simulink model "test_track1"  (R2023a)
settings: Solver=VariableStepAuto  StartTime=0.0  StopTime=600  RelTol=1e-3
settings Model: Creator=lpb10197  LastModifiedBy=lpb10197
settings DebuggingCC: UnconnectedInputMsg=warning  UnconnectedOutputMsg=warning  UnconnectedLineMsg=warning
settings ModelReferenceCC: EnableRefExpFcnMdlSchedulingChecks=on
settings RTWCC: DLArmComputeVersion=19.05

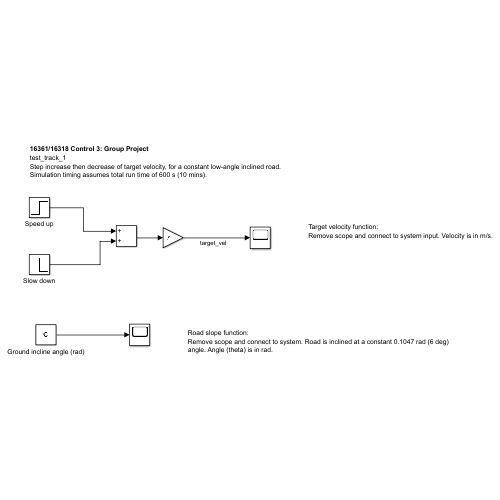
[thumbnail: Simulink's stored preview of the top-level diagram]
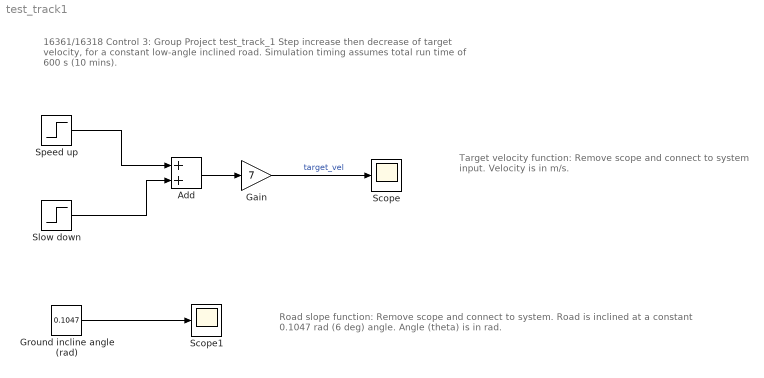
== system test_track1 ==
  note: Road slope function:
      | Remove scope and connect to system. Road is inclined at a constant 0.1047 rad (6 deg) angle. Angle (theta) is in rad.
  note: Target velocity function:
      | Remove scope and connect to system input. Velocity is in m/s.
  note: 16361/16318 Control 3: Group Project
      | test_track_1
      | Step increase then decrease of target velocity, for a constant low-angle inclined road.
      | Simulation timing assumes total run time of 600 s (10 mins).
  Add : Sum
  Gain : Gain  Gain=7
  Ground incline angle (rad) : Constant  Value=0.1047
  Scope : Scope
  Scope1 : Scope
  Slow down : Step  Time=300  Before=3  After=2  SampleTime=0
  Speed up : Step  Time=50  Before=1  After=3  SampleTime=0
  wires:
  Speed up/1 -> Add/1
  Slow down/1 -> Add/2
  Add/1 -> Gain/1
  Gain/1 -> Scope/1  "target_vel"
  Ground incline angle (rad)/1 -> Scope1/1
